simulink model "scenario_2_TIV_test_R2019a"  (R2019a)
settings: Solver=FixedStepAuto  StartTime=0.0  StopTime=60.0  FixedStep=1e-2  RelTol=1e-3
libraries: simulink x1
settings Model: Creator=Admin  LastModifiedBy=Admin

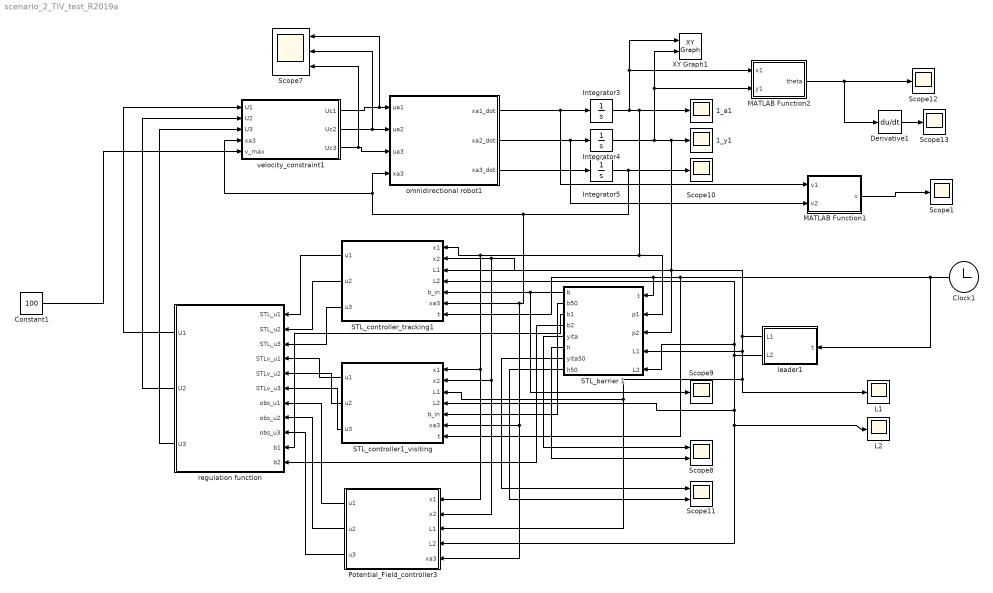
== system scenario_2_TIV_test_R2019a ==
  1_a1 : Scope
  1_y1 : Scope
  Clock1 : Clock
  Constant1 : Constant  Value=100
  Derivative1 : Derivative
  Integrator3 : Integrator
  Integrator4 : Integrator  InitialCondition=5
  Integrator5 : Integrator
  L1 : Scope
  L2 : Scope
  MATLAB Function1 : MATLAB Function  TreatAsAtomicUnit=on
  MATLAB Function2 : MATLAB Function  TreatAsAtomicUnit=on
  Potential_Field_controller3 : MATLAB Function  TreatAsAtomicUnit=on
  STL_barrier 1 : MATLAB Function  TreatAsAtomicUnit=on
  STL_controller1_visiting : MATLAB Function  TreatAsAtomicUnit=on
  STL_controller_tracking1 : MATLAB Function  TreatAsAtomicUnit=on
  Scope{1,9..10,12..13} (5 alike) : Scope
  Scope11 : Scope  NumInputPorts=2
  Scope7 : Scope  NumInputPorts=3
  Scope8 : Scope  NumInputPorts=2
  XY Graph1 : simulink/Sinks/XY Graph  xmin=-60  xmax=60  ymin=-60  ymax=60  st=0.01
  leader1 : MATLAB Function  TreatAsAtomicUnit=on
  omnidirectional robot1 : MATLAB Function  TreatAsAtomicUnit=on
  "regulation function " : MATLAB Function  TreatAsAtomicUnit=on
  velocity_constraint1 : MATLAB Function  TreatAsAtomicUnit=on
  wires:
  STL_barrier 1/6(h) -> Scope8/2
  Integrator3/1 -> MATLAB Function2/1(x1), XY Graph1/1, STL_barrier 1/2(p1), Potential_Field_controller3/1(x1), STL_controller1_visiting/1(x1), STL_controller_tracking1/1(x1), 1_a1/1
  leader1/2(L2) -> STL_barrier 1/5(L2), STL_controller_tracking1/4(L2), Potential_Field_controller3/4(L2), L2/1, STL_controller1_visiting/4(L2)
  STL_barrier 1/4(b2) -> "regulation function "/11(b2)
  Potential_Field_controller3/3(u3) -> "regulation function "/9(obs_u3)
  velocity_constraint1/1(Uc1) -> Scope7/1, omnidirectional robot1/1(ua1)
  omnidirectional robot1/3(xa3_dot) -> Integrator5/1
  Clock1/1 -> STL_barrier 1/1(t), STL_controller_tracking1/7(t), STL_controller1_visiting/7(t), leader1/1(t)
  velocity_constraint1/3(Uc3) -> Scope7/3, omnidirectional robot1/3(ua3)
  STL_barrier 1/5(yita) -> Scope8/1
  Constant1/1 -> velocity_constraint1/5(v_max)
  MATLAB Function2/1(theta) -> Derivative1/1, Scope12/1
  STL_controller_tracking1/3(u3) -> "regulation function "/3(STL_u3)
  Potential_Field_controller3/1(u1) -> "regulation function "/7(obs_u1)
  STL_barrier 1/3(b1) -> "regulation function "/10(b1)
  STL_barrier 1/8(h50) -> Scope11/2
  STL_barrier 1/2(b50) -> STL_controller1_visiting/5(b_in)
  velocity_constraint1/2(Uc2) -> Scope7/2, omnidirectional robot1/2(ua2)
  leader1/1(L1) -> STL_barrier 1/4(L1), L1/1, Potential_Field_controller3/3(L1), STL_controller1_visiting/3(L1), STL_controller_tracking1/3(L1)
  Integrator4/1 -> MATLAB Function2/2(y1), XY Graph1/2, STL_barrier 1/3(p2), Potential_Field_controller3/2(x2), STL_controller1_visiting/2(x2), STL_controller_tracking1/2(x2), 1_y1/1
  "regulation function "/3(U3) -> velocity_constraint1/3(U3)
  STL_barrier 1/1(b) -> Scope9/1, STL_controller_tracking1/5(b_in)
  omnidirectional robot1/1(xa1_dot) -> MATLAB Function1/1(v1), Integrator3/1
  "regulation function "/2(U2) -> velocity_constraint1/2(U2)
  omnidirectional robot1/2(xa2_dot) -> MATLAB Function1/2(v2), Integrator4/1
  "regulation function "/1(U1) -> velocity_constraint1/1(U1)
  Integrator5/1 -> velocity_constraint1/4(xa3), omnidirectional robot1/4(xa3), Potential_Field_controller3/5(xa3), STL_controller1_visiting/6(xa3), STL_controller_tracking1/6(xa3), Scope10/1
  STL_barrier 1/7(yita50) -> Scope11/1
  STL_controller_tracking1/2(u2) -> "regulation function "/2(STL_u2)
  STL_controller1_visiting/3(u3) -> "regulation function "/6(STLv_u3)
  Potential_Field_controller3/2(u2) -> "regulation function "/8(obs_u2)
  Derivative1/1 -> Scope13/1
  STL_controller1_visiting/2(u2) -> "regulation function "/5(STLv_u2)
  STL_controller_tracking1/1(u1) -> "regulation function "/1(STL_u1)
  STL_controller1_visiting/1(u1) -> "regulation function "/4(STLv_u1)
  MATLAB Function1/1(v) -> Scope1/1

== matlab function scenario_2_TIV_test_R2019a/MATLAB Function1 ==
  data: v1 input; v output; v2 input
function v = fcn(v1, v2)
v=sqrt(v1^2+v2^2);

== matlab function scenario_2_TIV_test_R2019a/MATLAB Function2 ==
  data: x1 input; theta output; y1 input
function theta = fcn(x1, y1)
theta=atan2(y1,x1);

== matlab function scenario_2_TIV_test_R2019a/Potential_Field_controller3 ==
  data: x1 input; x2 input; L1 input; L2 input; u1 output; xa3 input; u2 output; u3 output
function [u1,u2,u3] = fcn(x1, x2,L1,L2, xa3)
coder.extrinsic('Calculate_gradient');
coder.extrinsic('Calculate_gradient_x15');
coder.extrinsic('PVF_optimizer');
coder.extrinsic('add_random');
A1=[-1,0;0,-1];
F=[2*L1,2*L2];
distance=sqrt((x1-90)^2+(x2-90)^2);

gradient_x=0;gradient_y=0;
gradient_x5=0;gradient_y5=0;
[gradient_x,gradient_y]=Calculate_gradient(x1,x2,A1,F,0,30,8);
% gradient_x=Gradient(1,1);
% gradient_y=Gradient(1,2);
gradient_z=0;

Gradient_all=[gradient_x;gradient_y;gradient_z];
Li=0.2;
Bi=[0,cos(pi/6),-cos(pi/6);
    -1,sin(pi/6),sin(pi/6);
    Li,Li,Li;];

R1=[cos(xa3),-sin(xa3),0;
    sin(xa3),cos(xa3),0;
    0,0,1;];
R=0.02;
gx=R1*inv(Bi')*R;
A=Gradient_all'*gx;

%H=[1];
%H=[1,0;0,1];
%H=[0,0,0;0,0,0;0,0,0];
% H=[1,0,0;0,1,0;0,0,1];
 H=(1/2)*gx'*gx;
b=[0];
F=[-2*gx'*20*Gradient_all];
%=[];
u1=0;u2=0;u3=0;
U=PVF_optimizer(H,b,A,F,distance,gradient_x,gradient_y);

u1=U(1,1);
u2=U(2,1);
u3=U(3,1);

== matlab function scenario_2_TIV_test_R2019a/STL_barrier 1 ==
  data: b output; b50 output; b1 output; b2 output; yita output; h output; t input; p1 input; p2 input; L1 input; L2 input; yita50 output; h50 output
function [b,b50,b1,b2,yita,h,yita50,h50] = fcn(t,p1,p2,L1,L2)
d1=L1;
d2=L2;

d11=50;
d22=0;

d111=0;d222=30;

b=25*exp(-0.32*t)+5-sqrt( (p1-d1)^2 + (p2-d2)^2 ); %STL_tracking
yita=-25*exp(-0.32*t)+10;
h=15-sqrt( (p1-d1)^2 + (p2-d2)^2 );


b50=60*exp(-0.125*(t))+5-sqrt( (p1-d11)^2 + (p2-d22)^2 );%STL_visiting 
yita50=-60*exp(-0.125*(t))+5;
h50=10-sqrt( (p1-d11)^2 + (p2-d22)^2 );


% b50=5-sqrt( (p1-d11)^2 + (p2-d22)^2 );
% yita50=5;
% h50=10-sqrt( (p1-d11)^2 + (p2-d22)^2 );

b1=sqrt( (p1-d11)^2 + (p2-d22)^2 )-0;%STL_visiting_trigger

b21=sqrt( (p1-d111)^2 + (p2-d222)^2 )-6;
% b22=sqrt( (p1-agent5_x1)^2 + (p2-agent5_x2)^2 )-6;
b2=-(1/20)*log(exp(-20*b21)); %obstacle_avoidence_trigger

== matlab function scenario_2_TIV_test_R2019a/STL_controller1_visiting ==
  data: x1 input; x2 input; L1 input; L2 input; b_in input; u1 output; xa3 input; u2 output; u3 output; t input
function [u1,u2,u3]= fcn(x1, x2,L1,L2, b_in, xa3,t)
coder.extrinsic('quadoptimizer');
%coder.extrinsic('save');
d1=50; d2=0;

partial_b=(1/2)*((x1-d1)^2+(x2-d2)^2)^(-1/2);
partial_b_x=[-2*partial_b*(x1-d1),-2*partial_b*(x2-d2),0];


Li=0.2;
Bi=[0,cos(pi/6),-cos(pi/6);
    -1,sin(pi/6),sin(pi/6);
    Li,Li,Li;];

R1=[cos(xa3),-sin(xa3),0;
    sin(xa3),cos(xa3),0;
    0,0,1;];
R=0.02;

gx=R1*inv(Bi')*R;

A=partial_b_x*gx;

H=[1,0,0;0,1,0;0,0,1];
%H=[1];

b=150*b_in-0.125*60*exp(-0.125*(t))-50;

%  b=500*b_in-50;


u1=0;u2=0;u3=0;
U=quadoptimizer(H,b,A);

%U=quadprod(H,[],-A,b);

u1=U(1,1);
u2=U(2,1);
u3=U(3,1);

== matlab function scenario_2_TIV_test_R2019a/STL_controller_tracking1 ==
  data: x1 input; x2 input; L1 input; L2 input; b_in input; u1 output; xa3 input; u2 output; u3 output; t input
function [u1,u2,u3]= fcn(x1, x2,L1,L2, b_in, xa3,t)
coder.extrinsic('quadoptimizer');
%coder.extrinsic('save');
d1=L1; d2=L2;

partial_b=(1/2)*((x1-d1)^2+(x2-d2)^2)^(-1/2);
partial_b_x=[-2*partial_b*(x1-d1),-2*partial_b*(x2-d2),0];
partial_b_L=[2*partial_b*(x1-d1),2*partial_b*(x2-d2)];
pho1=sqrt(partial_b_L(1,1)^2+partial_b_L(1,2)^2);
Li=0.2;
Bi=[0,cos(pi/6),-cos(pi/6);
    -1,sin(pi/6),sin(pi/6);
    Li,Li,Li;];

R1=[cos(xa3),-sin(xa3),0;
    sin(xa3),cos(xa3),0;
    0,0,1;];
R=0.02;

gx=R1*inv(Bi')*R;

A=partial_b_x*gx;

H=[1,0,0;0,1,0;0,0,1];
%H=[1];

% b=200*b_in-0.37*25*exp(-0.37*t)-300-30*pho1;
b=200*b_in-0.32*25*exp(-0.32*t)-300-30*pho1;


u1=0;u2=0;u3=0;
U=quadoptimizer(H,b,A);

%U=quadprod(H,[],-A,b);

u1=U(1,1);
u2=U(2,1);
u3=U(3,1);

== matlab function scenario_2_TIV_test_R2019a/leader1 ==
  data: t input; L1 output; L2 output
function [L1,L2] = fcn(t)
L1=30*sin(1*t);
L2=30*cos(1*t);

== matlab function scenario_2_TIV_test_R2019a/omnidirectional robot1 ==
  data: ua1 input; xa1_dot output; ua2 input; ua3 input; xa3 input; xa2_dot output; xa3_dot output
function [xa1_dot,xa2_dot,xa3_dot]= fcn(ua1,ua2,ua3,xa3)

Li=0.2;
Bi=[0,cos(pi/6),-cos(pi/6);
    -1,sin(pi/6),sin(pi/6);
    Li,Li,Li;];

R1=[cos(xa3),-sin(xa3),0;
    sin(xa3),cos(xa3),0;
    0,0,1;];
R=0.02;

A=R1*inv(Bi')*R*[ua1;ua2;ua3];
xa1_dot=A(1,1);
xa2_dot=A(2,1);
xa3_dot=A(3,1);

== matlab function scenario_2_TIV_test_R2019a/regulation function  ==
  data: STL_u1 input; U1 output; STL_u2 input; STL_u3 input; STLv_u1 input; STLv_u2 input; STLv_u3 input; obs_u1 input; obs_u2 input; obs_u3 input; b1 input; U2 output; U3 output; b2 input
function [U1,U2,U3] = fcn(STL_u1,STL_u2,STL_u3,STLv_u1,STLv_u2,STLv_u3,obs_u1,obs_u2,obs_u3,b1,b2)
U_track=[STL_u1;STL_u2;STL_u3];
U_visit=[STLv_u1;STLv_u2;STLv_u3];
U_obs=[obs_u1;obs_u2;obs_u3];

k=0.065;
lambda=1-exp(-k*max(b1,0));
U_goal=lambda*U_track+(1-lambda)*U_visit;
% U_goal=[0;0;0];
% U_goal=U_track;
j=0.15;
gamma=1-exp(-j*max(b2,0));
U=gamma*U_goal+(1-gamma)*U_obs;

% U=U_goal;
U1=0;U2=0;U3=0;
U1=U(1,1);
U2=U(2,1);
U3=U(3,1);

== matlab function scenario_2_TIV_test_R2019a/velocity_constraint1 ==
  data: U1 input; Uc1 output; U2 input; U3 input; xa3 input; v_max input; Uc2 output; Uc3 output
function [Uc1,Uc2,Uc3] = fcn(U1,U2,U3,xa3,v_max)

Li=0.2;
Bi=[0,cos(pi/6),-cos(pi/6);
    -1,sin(pi/6),sin(pi/6);
    Li,Li,Li;];

R1=[cos(xa3),-sin(xa3),0;
    sin(xa3),cos(xa3),0;
    0,0,1;];
R=0.02;
gx=R1*inv(Bi')*R;

U=[U1;U2;U3];
V=[0;0;0];
V=gx*U;
if V(1,1)^2+V(2,1)^2<=v_max^2
     U(1,1)= U(1,1);
     U(2,1)= U(2,1);
else 
    U(1,1)=sqrt(v_max^2/(V(1,1)^2+V(2,1)^2))*U(1,1);
    U(2,1)=sqrt(v_max^2/(V(1,1)^2+V(2,1)^2))*U(2,1);
    U(3,1)=sqrt(v_max^2/(V(1,1)^2+V(2,1)^2))*U(3,1);
end

Uc1=U(1,1);
Uc2=U(2,1);
Uc3=U(3,1);
